simulink model "tempCtrlTest"  (R2022a)
settings: Solver=VariableStepAuto  StartTime=0.0  StopTime=timeExp(end)  RelTol=1e-3
values from neighbouring files (symbols this model uses):
  ctrl = fltCtrl    [tempCtrlTest_ts.m]
libraries: filteredPIDController_ul x3
settings Model: Creator=Ayaz  LastModifiedBy=lhill8
settings SolverCC: AlgebraicLoopSolver=TrustRegion
settings DebuggingCC: UnconnectedInputMsg=warning  UnconnectedOutputMsg=warning  UnconnectedLineMsg=warning  SFMachineParentedDataDiag=warning  ArithmeticOperatorsInVariantConditions=warning
settings SFSimCC: CustomCodeUndefinedFunction=UseInterfaceOnly

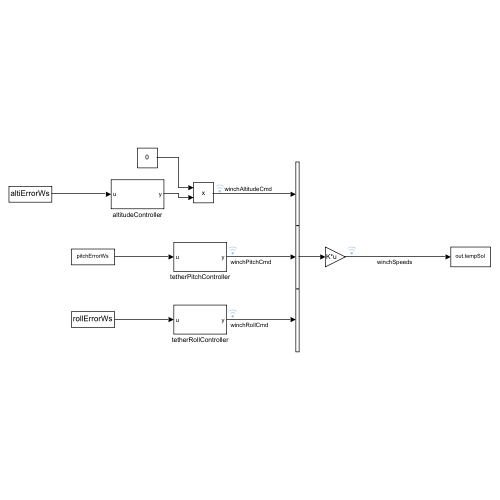
[thumbnail: Simulink's stored preview of the top-level diagram]
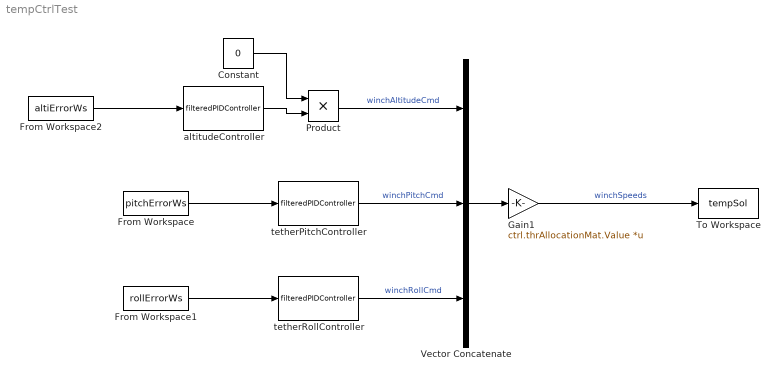
== system tempCtrlTest ==
  Constant : Constant  Value=0
  From Workspace : FromWorkspace  VariableName=pitchErrorWs
  From Workspace1 : FromWorkspace  VariableName=rollErrorWs
  From Workspace2 : FromWorkspace  VariableName=altiErrorWs
  Gain1 : Gain  Gain=ctrl.thrAllocationMat.Value  Multiplication=Matrix(K*u)
  Product : Product
  To Workspace : ToWorkspace  VariableName=tempSol  SaveFormat=Timeseries  SampleTime=-1
  Vector Concatenate : Concatenate  NumInputs=3
  altitudeController : filteredPIDController_ul/filteredPIDController  kp=ctrl.tetherAlti.kp.Value  ki=ctrl.tetherAlti.ki.Value  kd=ctrl.tetherAlti.kd.Value  Value=ctrl.tetherAlti.tau.Value  externalReset=none
  tetherPitchController : filteredPIDController_ul/filteredPIDController  kp=ctrl.tetherPitch.kp.Value  ki=ctrl.tetherPitch.ki.Value  kd=ctrl.tetherPitch.kd.Value  Value=ctrl.tetherPitch.tau.Value  externalReset=none
  tetherRollController : filteredPIDController_ul/filteredPIDController  kp=ctrl.tetherRoll.kp.Value  ki=ctrl.tetherRoll.ki.Value  kd=ctrl.tetherRoll.kd.Value  Value=ctrl.tetherRoll.tau.Value  externalReset=none
  wires:
  tetherPitchController/1 -> Vector Concatenate/2  "winchPitchCmd"
  Vector Concatenate/1 -> Gain1/1
  From Workspace1/1 -> tetherRollController/1
  Gain1/1 -> To Workspace/1  "winchSpeeds"
  From Workspace/1 -> tetherPitchController/1
  tetherRollController/1 -> Vector Concatenate/3  "winchRollCmd"
  From Workspace2/1 -> altitudeController/1
  Product/1 -> Vector Concatenate/1  "winchAltitudeCmd"
  altitudeController/1 -> Product/2
  Constant/1 -> Product/1
